simulink model "ssc_lithium_cell_2RC_laura_v7"  (R2021b)
settings: Solver=FixedStepAuto  StartTime=0.0  StopTime=t_sim_end  FixedStep=0.1  MaxStep=1  RelTol=1e-3  AbsTol=1e-3  EnableMultiTasking=on
PreLoadFcn:
  | ssc_lithium_cell_2RC_ini
values from neighbouring files (symbols this model uses):
  C1_LUT = [235.17 1246 1252.7 1261.4 1256.6 1258.7 1259.1 1259.8 1262.9 1235.3]    [IDprofile_mudle_25032022.m]    (also in Initialization.m = [1.2723e3 1.2723e3 1.2723e3 1.2723e3 1.2723e3 1.2723e3 1.272)
  C2_LUT = [90.935 3348.7 3590.5 3607.1 3645.6 3544.4 3532 3604.4 3591 4517.6]    [IDprofile_mudle_25032022.m]    (also in Initialization.m = [3.55e3 3.55e3 3.55e3 3.55e3 3.55e3 3.55e3 3.55e3 3.55e3 3.5)
  Cth = 25.95    [IDprofile_mudle_25032022.m]    (also in Initialization.m; Model_initialization5_SOC_solo.m)
  Em_LUT = [3.1658 3.4768 3.5975 3.7303 3.7706 3.7882 3.8381 3.9462 4.0582 4.1668]    [IDprofile_mudle_25032022.m]    (also in Initialization.m = interp1(SOC_full,Em_full,SOC_LUT); Model_initialization5_SOC_solo.m = interp1(SOC_full,Em_full,SOC_LUT))
  Ibat_test = Perfil_ID(1).I_A(435889:485758-3,1)    [IDprofile_mudle_25032022.m]    (also in Initialization.m; Model_initialization5_SOC_solo.m = Perfil_ID(3).I_A(354865+232:1607770+2700,1))
  Q0 = Q25/eff_45    [IDprofile_mudle_25032022.m]    (also in Initialization.m; Model_initialization5_SOC_solo.m = 1.3359)
  Qnom = Q25/eff_45    [IDprofile_mudle_25032022.m]    (also in Initialization.m; Model_initialization5_SOC_solo.m = 1.3359)
  R0_LUT = [0.0030829 0.072628 0.059416 0.043535 0.050516 0.04424 0.044157 0.042746 0.040859 0.035273]    [IDprofile_mudle_25032022.m]    (also in Initialization.m = [0.0024 0.0024 0.0024 0.0024 0.0024 0.0024 0.0024 0.0024 0.0)
  R1_LUT = [0.0015586 0.0052784 0.0076522 0.0073713 0.0040773 0.007966 0.0042052 0.0083473 0.0082109 0.0015675]    [IDprofile_mudle_25032022.m]    (also in Initialization.m = [0.0012 0.0012 0.0012 0.0012 0.0012 0.0012 0.0012 0.0012 0.0)
  R2_LUT = [0.010561 0.0057407 0.0077463 0.0090309 0.015808 0.0092643 0.0066197 0.030052 0.010592 0.0063853]    [IDprofile_mudle_25032022.m]    (also in Initialization.m = [0.0073 0.0073 0.0073 0.0073 0.0073 0.0073 0.0073 0.0073 0.0)
  Rcond = 0    [IDprofile_mudle_25032022.m]    (also in Initialization.m; Model_initialization5_SOC_solo.m)
  Rconv = 6.15    [IDprofile_mudle_25032022.m]    (also in Initialization.m; Model_initialization5_SOC_solo.m)
  SOC_LUT = linspace(SOC_full(1), SOC_full(end),10)    [IDprofile_mudle_25032022.m]    (also in Initialization.m; Model_initialization5_SOC_solo.m)
  T_init = 273.15 + 45 -1    (= 317.15)    [IDprofile_mudle_25032022.m]    (also in Initialization.m; Model_initialization5_SOC_solo.m = 318.15)
  Tbat_test = Perfil_ID(1).T_deg(435889:485758-3,1)+273.15    [IDprofile_mudle_25032022.m]    (also in Initialization.m; Model_initialization5_SOC_solo.m = Perfil_ID(3).T_deg(354865+232:1607770+2700,1)+273.15)
  Time_test = Perfil_ID(1).t_h(435889:485758-3,1)-min(Perfil_ID(1).t_h(435889:485758-3,1))    [IDprofile_mudle_25032022.m]    (also in Initialization.m; Model_initialization5_SOC_solo.m = Perfil_ID(3).t_h(354865+232:1607770+2700,1)-min(Perfil_ID(3))
  Vbat_test = Perfil_ID(1).V_V(435889:485758-3,1)    [IDprofile_mudle_25032022.m]    (also in Initialization.m; Model_initialization5_SOC_solo.m = Perfil_ID(3).V_V(354865+232:1607770+2700,1))
undefined symbols (not defined in the file or in its folder): Temperature_LUT
CloseFcn:
  | try,close(h1_ssc_lithium_cell_2RC),end
  | clear h1_ssc_lithium_cell_2RC
  | clear simlog_ssc_lithium_cell_2RC
Description:
  | Lithium Battery Cell - Two RC-Branch Equivalent Circuit
settings Model: Creator=The MathWorks, Inc.  LastModifiedBy=lauraoca
settings SolverCC: AlgebraicLoopSolver=TrustRegion
settings DataIOCC: LimitDataPoints=on  SaveFormat=Array  ReturnWorkspaceOutputsName=SDOSimTest_Log
settings OptimizationCC: LifeSpan=inf
settings DebuggingCC: AllowSymbolicDim=off  PregeneratedLibrarySubsystemCodeDiagnostic=none  SFUnexpectedBacktrackingDiag=warning  SFNoUnconditionalDefaultTransitionDiag=warning  SFExecutionAtInitializationDiag=none  SFMachineParentedDataDiag=warning  ArithmeticOperatorsInVariantConditions=warning
settings HardwareCC: ProdBitPerPointer=32  ProdBitPerSizeT=32  ProdBitPerPtrDiffT=32  ProdLargestAtomicFloat=None  ProdIntDivRoundTo=Undefined  ProdEndianess=Unspecified  ProdWordSize=32  ProdHWDeviceType=32-bit Generic
settings ModelReferenceCC: PropagateSignalLabelsOutOfModel=off
settings SFSimCC: SimUseLocalCustomCode=off  CustomCodeUndefinedFunction=UseInterfaceOnly
settings RTWCC: RTWUseLocalCustomCode=off
settings CodeAppCC: StateflowObjectComments=on
settings GRTTargetCC: TargetLangStandard=C89/C90 (ANSI)
settings ConfigComp: CovMetricSettings=dw  CovSaveCumulativeToWorkspaceVar=on  CovSaveSingleToWorkspaceVar=on  CovExternalEMLEnable=off  CovSFcnEnable=off
settings SimscapeCC: SimscapeLogType=all  SimscapeLogSimulationStatistics=on  SimscapeLogName=simlog_ssc_lithium_cell_2RC  SimscapeLogDataHistory=10000

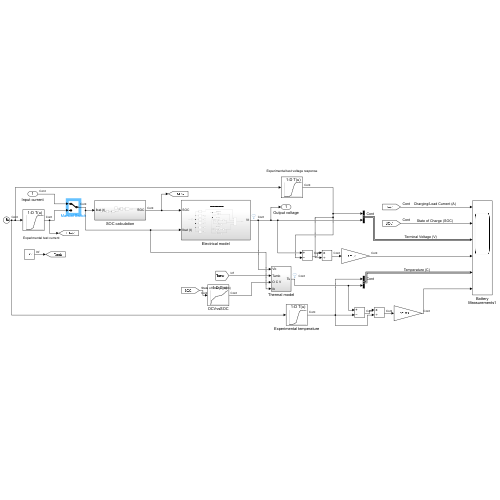
[thumbnail: Simulink's stored preview of the top-level diagram]
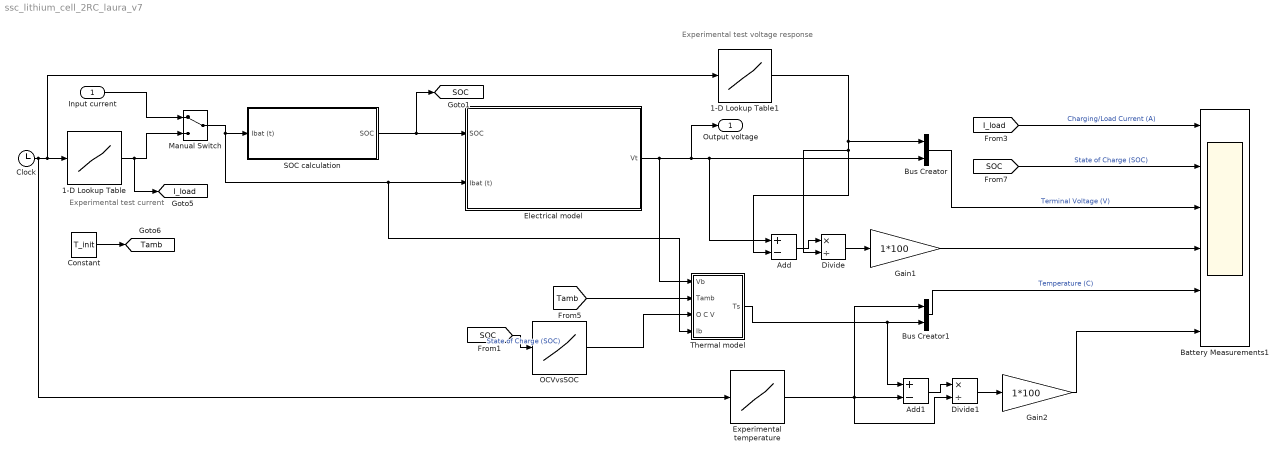
== system ssc_lithium_cell_2RC_laura_v7 ==
  note: Experimental test voltage response
  note: Experimental test current
  Input current : Inport
  1-D Lookup Table : Lookup_n-D  NumberOfTableDimensions=1  BreakpointsForDimension1=Time_test  Table=Ibat_test  InternalRulePriority=Speed  RndMeth=Simplest  InputSameDT=on
  1-D Lookup Table1 : Lookup_n-D  NumberOfTableDimensions=1  BreakpointsForDimension1=Time_test  Table=Vbat_test  InternalRulePriority=Speed  RndMeth=Simplest  InputSameDT=on
  Add : Sum  Inputs=+-
  Add1 : Sum  Inputs=+-
  Battery Measurements1 : Scope  NumInputPorts=6
  Bus Creator : BusCreator  Inputs=2
  Bus Creator1 : BusCreator  Inputs=2
  Clock : Clock
  Constant : Constant  Value=T_init
  Divide : Product  Inputs=*/
  Divide1 : Product  Inputs=*/
  Electrical model : Subsystem
  Experimental temperature : Lookup_n-D  NumberOfTableDimensions=1  BreakpointsForDimension1=Time_test  Table=Tbat_test  InternalRulePriority=Speed  RndMeth=Simplest  InputSameDT=on
  Gain1 : Gain  Gain=1*100
  Gain2 : Gain  Gain=1*100
  Manual Switch : ManualSwitch
  OCVvsSOC : Lookup_n-D  NumberOfTableDimensions=1  BreakpointsForDimension1=SOC_LUT  BreakpointsForDimension2=Temperature_LUT  Table=Em_LUT  InternalRulePriority=Speed  RndMeth=Simplest  InputSameDT=on
  SOC calculation : Subsystem
  Thermal model : Subsystem
  Output voltage : Outport  VectorParamsAs1DForOutWhenUnconnected=off
  tag scope: I_load=global, SOC=global, Tamb=global
  wires:
  SOC calculation/1(SOC) -> [SOC], Electrical model/1(SOC)
  Electrical model/1(Vt) -> Output voltage/1, Bus Creator/2, Add/1, Thermal model/1(Vb)
  Manual Switch/1 -> Thermal model/4(Ib), Electrical model/2(Ibat (t)), SOC calculation/1(Ibat (t))
  1-D Lookup Table/1 -> [I_load], Manual Switch/2
  Input current/1 -> Manual Switch/1
  Constant/1 -> [Tamb]
  OCVvsSOC/1 -> Thermal model/3(O C V)
  Clock/1 -> Experimental temperature/1, 1-D Lookup Table1/1, 1-D Lookup Table/1
  [Tamb] -> Thermal model/2(Tamb)
  Thermal model/1(Ts) -> Add1/1, Bus Creator1/2
  [I_load] -> Battery Measurements1/1  "Charging/Load Current (A)"
  [SOC] -> Battery Measurements1/2  "State of Charge (SOC)"
  Bus Creator1/1 -> Battery Measurements1/5  "Temperature (C)"
  Bus Creator/1 -> Battery Measurements1/3  "Terminal Voltage (V)"
  [SOC] -> OCVvsSOC/1  "State of Charge (SOC)"
  1-D Lookup Table1/1 -> Add/2, Divide/2, Bus Creator/1
  Divide/1 -> Gain1/1
  Add/1 -> Divide/1
  Experimental temperature/1 -> Divide1/2, Add1/2, Bus Creator1/1
  Gain1/1 -> Battery Measurements1/4
  Add1/1 -> Divide1/1
  Divide1/1 -> Gain2/1
  Gain2/1 -> Battery Measurements1/6

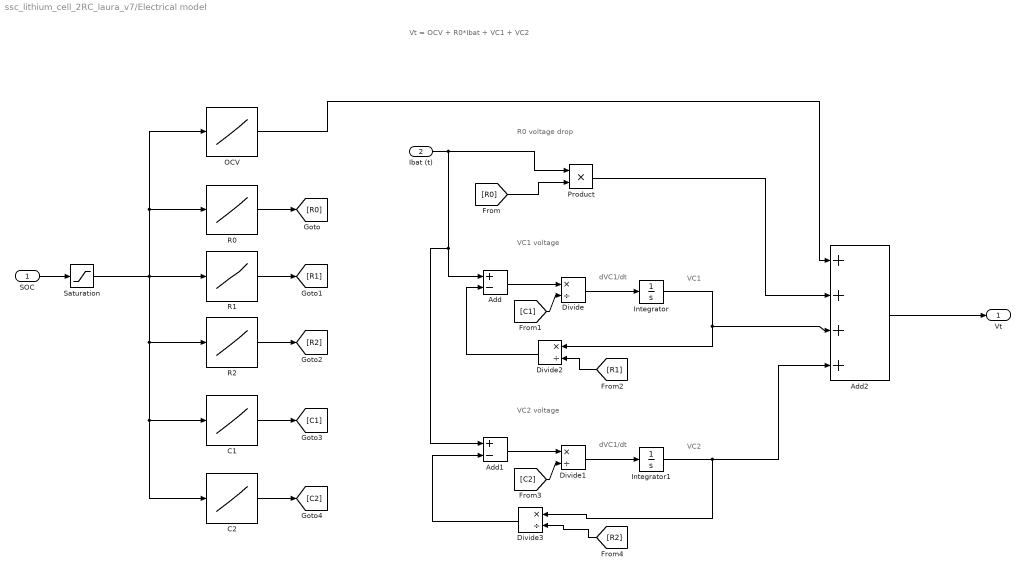
== system ssc_lithium_cell_2RC_laura_v7/Electrical model ==
  note: dVC1/dt
  note: VC1
  note: Vt = OCV + R0*Ibat + VC1 + VC2
  note: R0 voltage drop
  note: VC1 voltage
  note: dVC1/dt
  note: VC2
  note: VC2 voltage
  SOC : Inport
  Ibat (t) : Inport  Port=2
  Add : Sum  Inputs=+-
  Add1 : Sum  Inputs=+-
  Add2 : Sum  Inputs=++++
  C1 : Lookup_n-D  NumberOfTableDimensions=1  BreakpointsForDimension1=SOC_LUT  BreakpointsForDimension2=Temperature_LUT  Table=C1_LUT  InternalRulePriority=Speed  RndMeth=Simplest  InputSameDT=on
  C2 : Lookup_n-D  NumberOfTableDimensions=1  BreakpointsForDimension1=SOC_LUT  BreakpointsForDimension2=Temperature_LUT  Table=C2_LUT  InternalRulePriority=Speed  RndMeth=Simplest  InputSameDT=on
  Divide{,1..3} (4 alike) : Product  Inputs=*/
  Integrator : Integrator
  Integrator1 : Integrator
  OCV : Lookup_n-D  NumberOfTableDimensions=1  BreakpointsForDimension1=SOC_LUT  BreakpointsForDimension2=Temperature_LUT  Table=Em_LUT  InternalRulePriority=Speed  RndMeth=Simplest  InputSameDT=on
  Product : Product
  R0 : Lookup_n-D  NumberOfTableDimensions=1  BreakpointsForDimension1=SOC_LUT  BreakpointsForDimension2=Temperature_LUT  Table=R0_LUT  InternalRulePriority=Speed  RndMeth=Simplest  InputSameDT=on
  R1 : Lookup_n-D  NumberOfTableDimensions=1  BreakpointsForDimension1=SOC_LUT  BreakpointsForDimension2=Temperature_LUT  Table=R1_LUT  InternalRulePriority=Speed  RndMeth=Simplest  InputSameDT=on
  R2 : Lookup_n-D  NumberOfTableDimensions=1  BreakpointsForDimension1=SOC_LUT  BreakpointsForDimension2=Temperature_LUT  Table=R2_LUT  InternalRulePriority=Speed  RndMeth=Simplest  InputSameDT=on
  Saturation : Saturate  UpperLimit=SOC_LUT(10)  LowerLimit=SOC_LUT(1)
  Vt : Outport  VectorParamsAs1DForOutWhenUnconnected=off
  wires:
  C2/1 -> [C2]
  R0/1 -> [R0]
  R2/1 -> [R2]
  R1/1 -> [R1]
  C1/1 -> [C1]
  [R0] -> Product/2
  Add/1 -> Divide/1
  [C1] -> Divide/2
  Divide/1 -> Integrator/1
  Integrator/1 -> Divide2/1, Add2/3
  [R1] -> Divide2/2
  Divide2/1 -> Add/2
  Divide3/1 -> Add1/2
  [R2] -> Divide3/2
  Integrator1/1 -> Divide3/1, Add2/4
  Divide1/1 -> Integrator1/1
  [C2] -> Divide1/2
  Add1/1 -> Divide1/1
  Ibat (t)/1 -> Add1/1, Add/1, Product/1
  OCV/1 -> Add2/1
  Product/1 -> Add2/2
  Add2/1 -> Vt/1
  SOC/1 -> Saturation/1
  Saturation/1 -> C2/1, C1/1, R2/1, OCV/1, R0/1, R1/1

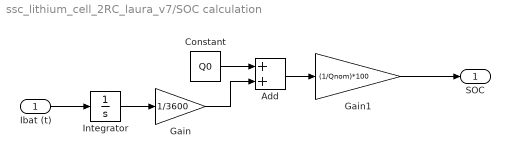
== system ssc_lithium_cell_2RC_laura_v7/SOC calculation ==
  Ibat (t) : Inport
  Add : Sum
  Constant : Constant  Value=Q0
  Gain : Gain  Gain=1/3600
  Gain1 : Gain  Gain=(1/Qnom)*100
  Integrator : Integrator
  SOC : Outport  VectorParamsAs1DForOutWhenUnconnected=off
  wires:
  Constant/1 -> Add/1
  Gain1/1 -> SOC/1
  Integrator/1 -> Gain/1
  Ibat (t)/1 -> Integrator/1
  Gain/1 -> Add/2
  Add/1 -> Gain1/1

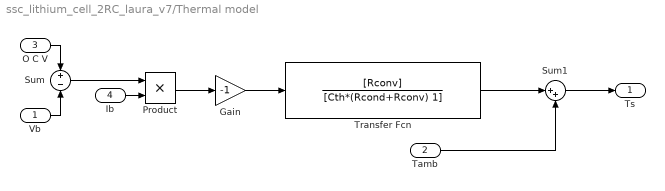
== system ssc_lithium_cell_2RC_laura_v7/Thermal model ==
  Vb : Inport
  Tamb : Inport  Port=2
  O C V : Inport  Port=3
  Ib : Inport  Port=4
  Gain : Gain  Gain=-1
  Product : Product
  Sum : Sum  Inputs=+|-
  Sum1 : Sum  Inputs=|++
  Transfer Fcn : TransferFcn  Numerator=[Rconv]  Denominator=[Cth*(Rcond+Rconv) 1]
  Ts : Outport
  wires:
  Tamb/1 -> Sum1/2
  Transfer Fcn/1 -> Sum1/1
  Sum1/1 -> Ts/1
  Sum/1 -> Product/1
  Product/1 -> Gain/1
  Gain/1 -> Transfer Fcn/1
  Vb/1 -> Sum/2
  O C V/1 -> Sum/1
  Ib/1 -> Product/2
